simulink model "thirdhormonicemfingection"  (R2022b)
settings: Solver=ode3  StartTime=0.0  StopTime=0.5  FixedStep=5e-5  RelTol=1e-3
libraries: spsIGBTDiodeLib x6, simulink x3, spsSeriesRLCBranchLib x3, spsVoltageMeasurementLib x2, spsDCVoltageSourceLib x1, spspowerguiLib x1
settings Model: Creator=gudel  LastModifiedBy=gudel

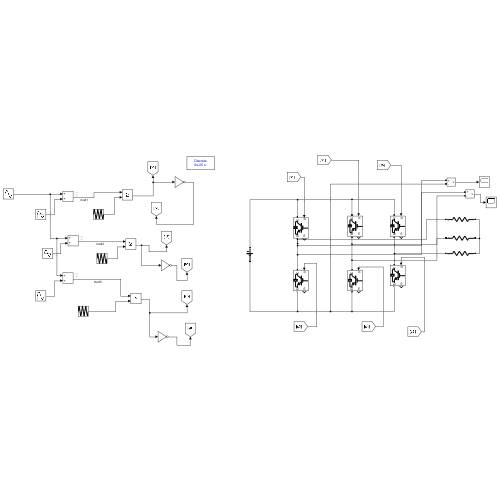
[thumbnail: Simulink's stored preview of the top-level diagram]
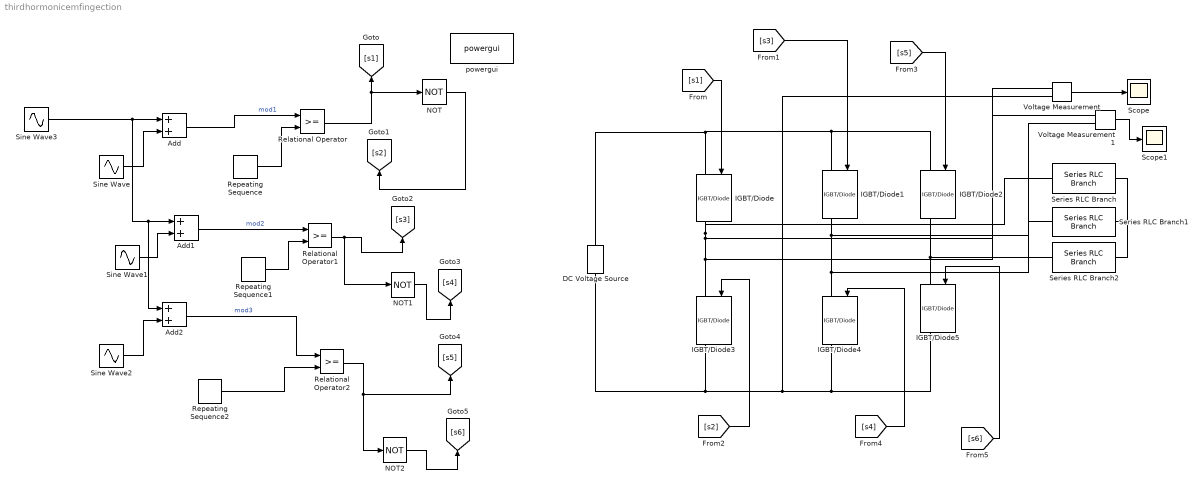
== system thirdhormonicemfingection ==
  Add : Sum
  Add1 : Sum
  Add2 : Sum
  DC Voltage Source : spsDCVoltageSourceLib/DC Voltage Source  Amplitude=100  Measurements=Voltage
  IGBT/Diode{,1..5} (6 alike) : spsIGBTDiodeLib/IGBT//Diode  Ron=1e-3  Rs=1e5  Cs=inf  Measurements=on
  NOT : Logic  Operator=NOT  IconShape=distinctive  AllPortsSameDT=off  OutDataTypeStr=boolean
  NOT1 : Logic  Operator=NOT  IconShape=distinctive  AllPortsSameDT=off  OutDataTypeStr=boolean
  NOT2 : Logic  Operator=NOT  IconShape=distinctive  AllPortsSameDT=off  OutDataTypeStr=boolean
  Relational Operator : RelationalOperator  OutDataTypeStr=boolean  RndMeth=Simplest  InputSameDT=off
  Relational Operator1 : RelationalOperator  OutDataTypeStr=boolean  RndMeth=Simplest  InputSameDT=off
  Relational Operator2 : RelationalOperator  OutDataTypeStr=boolean  RndMeth=Simplest  InputSameDT=off
  Repeating Sequence : simulink/Sources/Repeating Sequence  rep_seq_t=[0 0.25 0.5 0.75 1]*1/2000  rep_seq_y=[0 1 0 -1 0]
  Repeating Sequence1 : simulink/Sources/Repeating Sequence  rep_seq_t=[0 0.25 0.5 0.75 1]*1/2000  rep_seq_y=[0 1 0 -1 0]
  Repeating Sequence2 : simulink/Sources/Repeating Sequence  rep_seq_t=[0 0.25 0.5 0.75 1]*1/2000  rep_seq_y=[0 1 0 -1 0]
  Scope : Scope
  Scope1 : Scope
  Series RLC Branch : spsSeriesRLCBranchLib/Series RLC Branch  LConnTagsString=__new0  RConnTagsString=__new0  BranchType=R  Resistance=20  Inductance=1e-3  SetiL0=off  InitialCurrent=0  Capacitance=1e-6  Setx0=off  InitialVoltage=0  Measurements=None
  Series RLC Branch1 : spsSeriesRLCBranchLib/Series RLC Branch  LConnTagsString=__new0  RConnTagsString=__new0  BranchType=R  Resistance=20  Inductance=1e-3  SetiL0=off  InitialCurrent=0  Capacitance=1e-6  Setx0=off  InitialVoltage=0  Measurements=None
  Series RLC Branch2 : spsSeriesRLCBranchLib/Series RLC Branch  LConnTagsString=__new0  RConnTagsString=__new0  BranchType=R  Resistance=20  Inductance=1e-3  SetiL0=off  InitialCurrent=0  Capacitance=1e-6  Setx0=off  InitialVoltage=0  Measurements=None
  Sine Wave : Sin  Amplitude=1.15  Frequency=2*pi*50  SampleTime=0
  Sine Wave1 : Sin  Amplitude=1.15  Frequency=2*pi*50  Phase=[2/3]*pi  SampleTime=0
  Sine Wave2 : Sin  Amplitude=1.15  Frequency=2*pi*50  Phase=[4/3]*pi  SampleTime=0
  Sine Wave3 : Sin  Amplitude=1.15/6  Frequency=2*pi*50*3  SampleTime=0
  Voltage Measurement : spsVoltageMeasurementLib/Voltage Measurement  PhasorSimulation=off  OutputType=Complex  PSBequivalent=0
  Voltage Measurement1 : spsVoltageMeasurementLib/Voltage Measurement  PhasorSimulation=off  OutputType=Complex  PSBequivalent=0
  powergui : spspowerguiLib/powergui  Priority=1  SimulationMode=Discrete  SampleTime=50e-6  frequency=60  Iterations=50  frequencyindice=0  Pbase=100e6  ErrMax=1e-4  UnitsV=kV  UnitsW=MW  buscounter=0  FunctionMessages=off  echomessages=off  EnableUseOfTLC=off  CurrentSourceSwitches=off  DisableSnubberDevices=off  DisableRonSwitches=off  DisableVfSwitches=off  DisplayEquations=off  AutomaticDiscreteSolvers=off  SolverType=Tustin/Backward Euler (TBE)  Interpol=off  ExternalGateDelay=off  methode=off  Ts=100  x0status=blocks  SPID=on  SwTol=0  HookPort=off  NonlinearTolerance=1e-4  nMaxIteration=100  ContinueOnMaxIteration=off  RestoreLinks=warning  ResistiveCurrentMeasurement=off  Frange=[0:2:500]  Ylog=off  Xlog=on  ShowGrid=off  save=off  variable=ZData  structure=0  ZoomFFT=off  StartTime=0.0  cycles=1  DisplayStyle=1  fundamental=60  FreqAxis=off  MaxFrequency=1000  frequencyindicesteady=1  RmsSteady=1  display=off
  wires:
  Sine Wave3/1 -> Add2/1, Add1/1, Add/1
  Sine Wave/1 -> Add/2
  Sine Wave2/1 -> Add2/2
  Sine Wave1/1 -> Add1/2
  Repeating Sequence/1 -> Relational Operator/2
  Add/1 -> Relational Operator/1  "mod1"
  Add1/1 -> Relational Operator1/1  "mod2"
  Repeating Sequence1/1 -> Relational Operator1/2
  Repeating Sequence2/1 -> Relational Operator2/2
  Add2/1 -> Relational Operator2/1  "mod3"
  Relational Operator/1 -> NOT/1, [s1]
  NOT/1 -> [s2]
  Relational Operator1/1 -> NOT1/1, [s3]
  NOT1/1 -> [s4]
  NOT2/1 -> [s6]
  Relational Operator2/1 -> [s5], NOT2/1
  [s1] -> IGBT/Diode/1
  [s3] -> IGBT/Diode1/1
  [s2] -> IGBT/Diode3/1
  [s4] -> IGBT/Diode4/1
  [s6] -> IGBT/Diode5/1
  [s5] -> IGBT/Diode2/1
  Voltage Measurement/1 -> Scope/1
  Voltage Measurement1/1 -> Scope1/1
  connections:
  IGBT/Diode3/RConn1 -- Voltage Measurement/LConn2 -- IGBT/Diode4/RConn1 -- IGBT/Diode5/RConn1 -- DC Voltage Source/LConn1
  IGBT/Diode/RConn1 -- Voltage Measurement/LConn1 -- Voltage Measurement1/LConn1 -- IGBT/Diode3/LConn1 -- Series RLC Branch/LConn1
  IGBT/Diode1/RConn1 -- Voltage Measurement1/LConn2 -- IGBT/Diode4/LConn1 -- Series RLC Branch1/LConn1
  IGBT/Diode2/RConn1 -- Series RLC Branch2/LConn1 -- IGBT/Diode5/LConn1
  IGBT/Diode/LConn1 -- DC Voltage Source/RConn1 -- IGBT/Diode1/LConn1 -- IGBT/Diode2/LConn1
  Series RLC Branch/RConn1 -- Series RLC Branch1/RConn1 -- Series RLC Branch2/RConn1
